simulink model "ActatorValidation"  (R2024b)
settings: Solver=VariableStepAuto  StartTime=0.0  StopTime=10.0  RelTol=1e-3
undefined symbols (not defined in the file): Aero
settings Model: Creator=Tyler  LastModifiedBy=Tyler

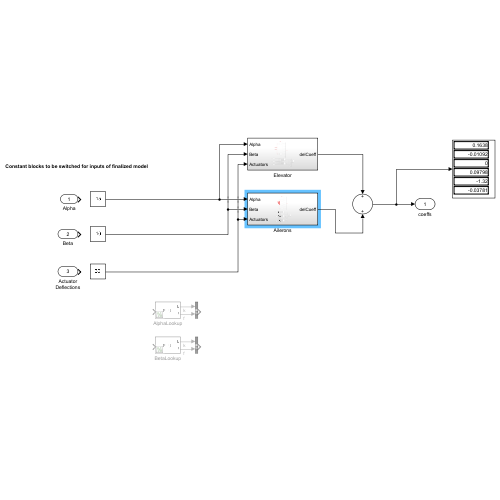
[thumbnail: Simulink's stored preview of the top-level diagram]
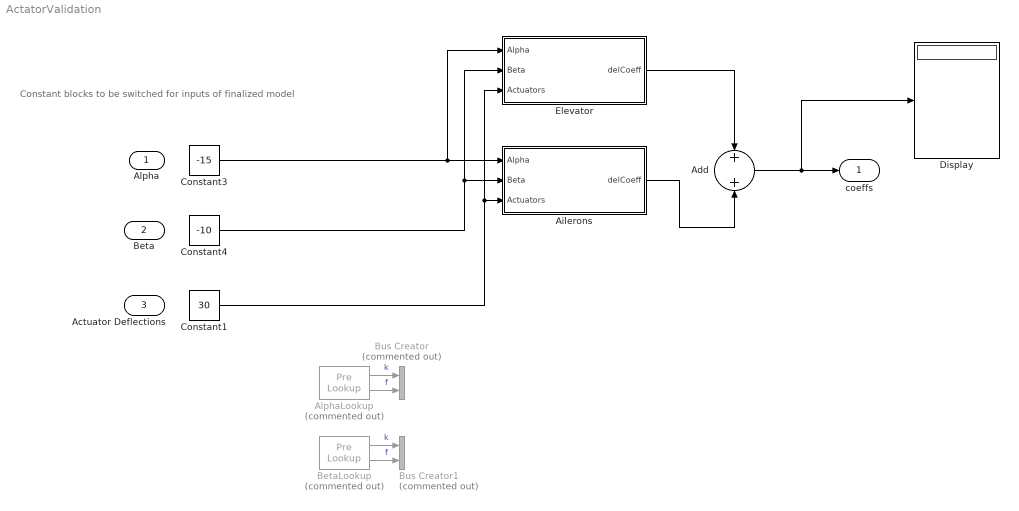
== system ActatorValidation ==
  note: Constant blocks to be switched for inputs of finalized model
  Alpha : Inport  Unit=deg
  Beta : Inport  Port=2  Unit=deg
  "Actuator Deflections " : Inport  Port=3
  Add : Sum
  Ailerons : Subsystem
  AlphaLookup : PreLookup  Commented=on  BreakpointsData=Aero.alpha_vec  BeginIndexSearchUsingPreviousIndexResult=on  ExtrapMethod=Linear
  BetaLookup : PreLookup  Commented=on  BreakpointsData=Aero.beta_vec  BeginIndexSearchUsingPreviousIndexResult=on  ExtrapMethod=Linear
  Bus Creator : BusCreator  Commented=on  Inputs=2
  Bus Creator1 : BusCreator  Commented=on  Inputs=2
  Constant1 : Constant  Value=30
  Constant3 : Constant  Value=-15
  Constant4 : Constant  Value=-10
  Display : Display
  Elevator : Subsystem
  coeffs : Outport  VectorParamsAs1DForOutWhenUnconnected=off
  wires:
  Elevator/1(delCoeff) -> Add/1
  Constant4/1 -> Ailerons/2(Beta), Elevator/2(Beta)
  BetaLookup/1 -> Bus Creator1/1  "k"
  AlphaLookup/1 -> Bus Creator/1  "k"
  AlphaLookup/2 -> Bus Creator/2  "f"
  Constant1/1 -> Ailerons/3(Actuators), Elevator/3(Actuators)
  Ailerons/1(delCoeff) -> Add/2
  BetaLookup/2 -> Bus Creator1/2  "f"
  Add/1 -> Display/1, coeffs/1
  Constant3/1 -> Ailerons/1(Alpha), Elevator/1(Alpha)

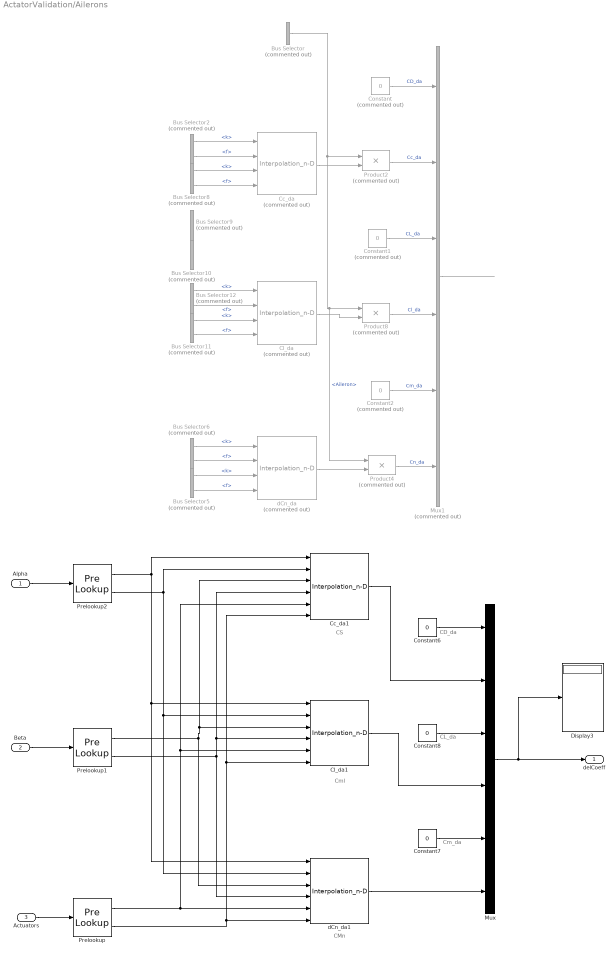
== system ActatorValidation/Ailerons ==
  note: CL_da
  note: CD_da
  note: Cm_da
  note: CMn
  note: CS
  note: Cml
  Alpha : Inport
  Beta : Inport  Port=2
  Actuators : Inport  Port=3
  Bus Selector : BusSelector  Commented=on  OutputSignals=Aileron
  Bus Selector{2,5..6,8..12} (8 alike) : BusSelector  Commented=on  OutputSignals=k,f
  Cc_da : Interpolation_n-D  Commented=on  Table=Aero.Cc_da  RemoveProtectionIndex=on  SaturateOnIntegerOverflow=on
  Cc_da1 : Interpolation_n-D  NumberOfTableDimensions=3  Table=Aero.Cc_da  RemoveProtectionIndex=on  SaturateOnIntegerOverflow=on
      settings: InputPortMap=u0,u1,u2,u3,u4,u5
  Cl_da : Interpolation_n-D  Commented=on  Table=Aero.Cl_da  RemoveProtectionIndex=on  SaturateOnIntegerOverflow=on
  Cl_da1 : Interpolation_n-D  NumberOfTableDimensions=3  Table=Aero.Cl_da  RemoveProtectionIndex=on  SaturateOnIntegerOverflow=on
      settings: InputPortMap=u0,u1,u2,u3,u4,u5
  Constant : Constant  Commented=on  Value=0
  Constant1 : Constant  Commented=on  Value=0
  Constant2 : Constant  Commented=on  Value=0
  Constant6 : Constant  Value=0
  Constant7 : Constant  Value=0
  Constant8 : Constant  Value=0
  Display3 : Display
  Mux : Mux  Inputs=6
  Mux1 : Mux  Commented=on  Inputs=6
  Prelookup : PreLookup  BreakpointsData=Aero.delta_vec  ExtrapMethod=Linear
  Prelookup1 : PreLookup  BreakpointsData=Aero.beta_vec  ExtrapMethod=Linear
  Prelookup2 : PreLookup  BreakpointsData=Aero.alpha_vec  ExtrapMethod=Linear
  Product2 : Product  Commented=on  InputSameDT=on  SaturateOnIntegerOverflow=on  OutDataTypeStr=Inherit: Same as first input
  Product4 : Product  Commented=on  InputSameDT=on  SaturateOnIntegerOverflow=on  OutDataTypeStr=Inherit: Same as first input
  Product8 : Product  Commented=on  InputSameDT=on  SaturateOnIntegerOverflow=on  OutDataTypeStr=Inherit: Same as first input
  dCn_da : Interpolation_n-D  Commented=on  Table=Aero.Cn_da  RemoveProtectionIndex=on  SaturateOnIntegerOverflow=on
  dCn_da1 : Interpolation_n-D  NumberOfTableDimensions=3  Table=Aero.Cn_da  RemoveProtectionIndex=on  SaturateOnIntegerOverflow=on
      settings: InputPortMap=u0,u1,u2,u3,u4,u5
  delCoeff : Outport  VectorParamsAs1DForOutWhenUnconnected=off
  wires:
  Cc_da/1 -> Product2/2
  Mux1/1 -> ?
  Product2/1 -> Mux1/2  "Cc_da"
  Bus Selector2/1 -> Cc_da/1  "<k>"
  ? -> Bus Selector/1
  Bus Selector2/2 -> Cc_da/2  "<f>"
  Constant/1 -> Mux1/1  "CD_da"
  Bus Selector8/1 -> Cc_da/3  "<k>"
  Bus Selector8/2 -> Cc_da/4  "<f>"
  Constant1/1 -> Mux1/3  "CL_da"
  Bus Selector11/2 -> Cl_da/4  "<f>"
  Bus Selector11/1 -> Cl_da/3  "<k>"
  Bus Selector12/2 -> Cl_da/2  "<f>"
  Bus Selector12/1 -> Cl_da/1  "<k>"
  Product8/1 -> Mux1/4  "Cl_da"
  Cl_da/1 -> Product8/2
  Bus Selector5/1 -> dCn_da/3  "<k>"
  ? -> Bus Selector5/1, Bus Selector11/1, Bus Selector10/1, Bus Selector8/1
  Bus Selector5/2 -> dCn_da/4  "<f>"
  dCn_da/1 -> Product4/2
  ? -> Bus Selector6/1, Bus Selector12/1, Bus Selector2/1, Bus Selector9/1
  Bus Selector6/2 -> dCn_da/2  "<f>"
  Bus Selector/1 -> Product4/1, Product8/1, Product2/1  "<Aileron>"
  Bus Selector6/1 -> dCn_da/1  "<k>"
  Constant2/1 -> Mux1/5  "Cm_da"
  Product4/1 -> Mux1/6  "Cn_da"
  Constant7/1 -> Mux/5
  Constant6/1 -> Mux/1
  dCn_da1/1 -> Mux/6
  Beta/1 -> Prelookup1/1
  Prelookup2/1 -> dCn_da1/1, Cl_da1/1, Cc_da1/1
  Cc_da1/1 -> Mux/2
  Mux/1 -> delCoeff/1, Display3/1
  Prelookup/1 -> Cc_da1/5, Cl_da1/5, dCn_da1/5
  Prelookup/2 -> Cc_da1/6, Cl_da1/6, dCn_da1/6
  Constant8/1 -> Mux/3
  Prelookup2/2 -> dCn_da1/2, Cl_da1/2, Cc_da1/2
  Cl_da1/1 -> Mux/4
  Prelookup1/2 -> Cc_da1/4, Cl_da1/4, dCn_da1/4
  Prelookup1/1 -> Cc_da1/3, Cl_da1/3, dCn_da1/3
  Actuators/1 -> Prelookup/1
  Alpha/1 -> Prelookup2/1

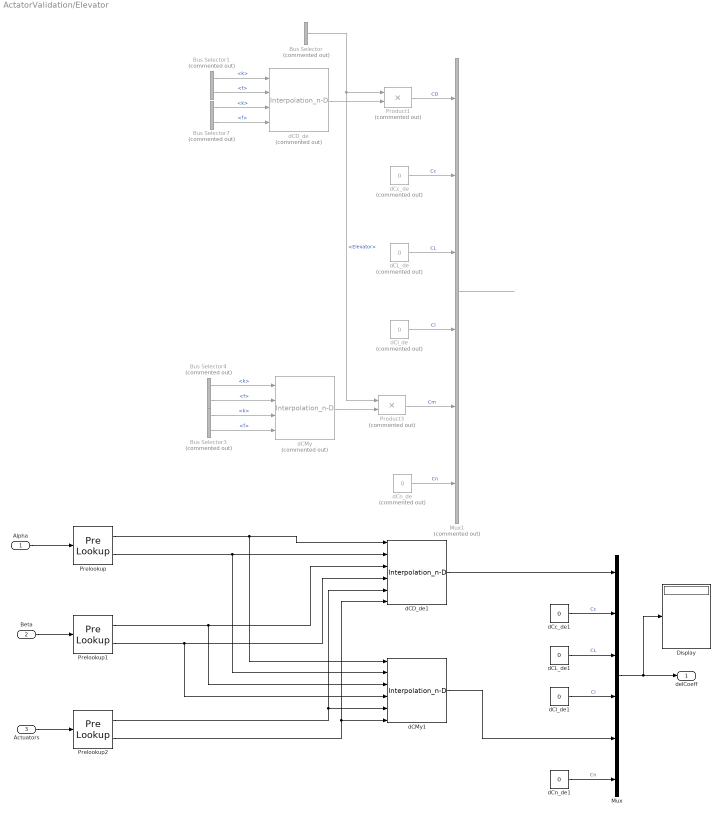
== system ActatorValidation/Elevator ==
  Alpha : Inport
  Beta : Inport  Port=2
  Actuators : Inport  Port=3
  Bus Selector : BusSelector  Commented=on  OutputSignals=Elevator
  Bus Selector{1,3..4,7} (4 alike) : BusSelector  Commented=on  OutputSignals=k,f
  Display : Display
  Mux : Mux  Inputs=6
  Mux1 : Mux  Commented=on  Inputs=6
  Prelookup : PreLookup  BreakpointsData=Aero.alpha_vec  ExtrapMethod=Linear
  Prelookup1 : PreLookup  BreakpointsData=Aero.beta_vec  ExtrapMethod=Linear
  Prelookup2 : PreLookup  BreakpointsData=Aero.delta_vec  ExtrapMethod=Linear
  Product1 : Product  Commented=on  InputSameDT=on  SaturateOnIntegerOverflow=on  OutDataTypeStr=Inherit: Same as first input
  Product3 : Product  Commented=on  InputSameDT=on  SaturateOnIntegerOverflow=on  OutDataTypeStr=Inherit: Same as first input
  dCD_de : Interpolation_n-D  Commented=on  Table=Aero.CD_de  RemoveProtectionIndex=on  SaturateOnIntegerOverflow=on
  dCD_de1 : Interpolation_n-D  NumberOfTableDimensions=3  Table=Aero.CD_de  RemoveProtectionIndex=on  SaturateOnIntegerOverflow=on
      settings: InputPortMap=u0,u1,u2,u3,u4,u5
  dCL_de : Constant  Commented=on  Value=0
  dCL_de1 : Constant  Value=0
  dCMy : Interpolation_n-D  Commented=on  Table=Aero.Cm_de  RemoveProtectionIndex=on  SaturateOnIntegerOverflow=on
  dCMy1 : Interpolation_n-D  NumberOfTableDimensions=3  Table=Aero.Cm_de  RemoveProtectionIndex=on  SaturateOnIntegerOverflow=on
      settings: InputPortMap=u0,u1,u2,u3,u4,u5
  dCc_de : Constant  Commented=on  Value=0
  dCc_de1 : Constant  Value=0
  dCl_de : Constant  Commented=on  Value=0
  dCl_de1 : Constant  Value=0
  dCn_de : Constant  Commented=on  Value=0
  dCn_de1 : Constant  Value=0
  delCoeff : Outport  VectorParamsAs1DForOutWhenUnconnected=off
  wires:
  Mux1/1 -> ?
  Bus Selector1/2 -> dCD_de/2  "<f>"
  dCc_de/1 -> Mux1/2  "Cc"
  ? -> Bus Selector/1
  dCD_de/1 -> Product1/2
  Bus Selector1/1 -> dCD_de/1  "<k>"
  Product1/1 -> Mux1/1  "CD"
  Bus Selector7/1 -> dCD_de/3  "<k>"
  Bus Selector7/2 -> dCD_de/4  "<f>"
  dCl_de/1 -> Mux1/4  "Cl"
  Bus Selector3/1 -> dCMy/3  "<k>"
  Bus Selector3/2 -> dCMy/4  "<f>"
  dCMy/1 -> Product3/2
  Bus Selector4/2 -> dCMy/2  "<f>"
  Bus Selector4/1 -> dCMy/1  "<k>"
  ? -> Bus Selector3/1, Bus Selector7/1
  ? -> Bus Selector4/1, Bus Selector1/1
  Bus Selector/1 -> Product3/1, Product1/1  "<Elevator>"
  Product3/1 -> Mux1/5  "Cm"
  dCn_de/1 -> Mux1/6  "Cn"
  dCL_de/1 -> Mux1/3  "CL"
  dCMy1/1 -> Mux/5
  dCn_de1/1 -> Mux/6  "Cn"
  Prelookup1/2 -> dCMy1/4, dCD_de1/4
  Alpha/1 -> Prelookup/1
  Prelookup2/1 -> dCMy1/5, dCD_de1/5
  Prelookup2/2 -> dCD_de1/6, dCMy1/6
  Prelookup1/1 -> dCMy1/3, dCD_de1/3
  Prelookup/2 -> dCMy1/2, dCD_de1/2
  dCD_de1/1 -> Mux/1
  dCL_de1/1 -> Mux/3  "CL"
  Prelookup/1 -> dCMy1/1, dCD_de1/1
  dCl_de1/1 -> Mux/4  "Cl"
  Beta/1 -> Prelookup1/1
  Actuators/1 -> Prelookup2/1
  dCc_de1/1 -> Mux/2  "Cc"
  Mux/1 -> delCoeff/1, Display/1
